simulink model "state_space_all_model_reduce"  (R2018a)
settings: Solver=FixedStepAuto  StartTime=0.0  StopTime=3  FixedStep=tm  MaxStep=1e-4  RelTol=1e-5  AbsTol=1e-5
InitFcn:
  | SimulinkInit_linea_transmision
values from neighbouring files (symbols this model uses):
  Ad = sysd.A    [SimulinkInit_linea_transmision.m]
  ataque = 1    [SimulinkInit_linea_transmision.m]
  b = 4.91    [SimulinkInit_linea_transmision.m]
  Bd = sysd.B    [SimulinkInit_linea_transmision.m]
  Bdr = sysdr.B    [SimulinkInit_linea_transmision.m]
  C = 1    [SimulinkInit_linea_transmision.m]
  C1 = 22e-6    (= 2.2e-05)    [SimulinkInit_linea_transmision.m]
  c11 = 0.04    [SimulinkInit_linea_transmision.m]
  c12 = 0.04    [SimulinkInit_linea_transmision.m]
  c13 = 1.7    [SimulinkInit_linea_transmision.m]
  c14 = 0.17    [SimulinkInit_linea_transmision.m]
  C1o = Cd(2,:)    [SimulinkInit_linea_transmision.m]
  C2 = 22e-6    (= 2.2e-05)    [SimulinkInit_linea_transmision.m]
  c21 = 0.04    [SimulinkInit_linea_transmision.m]
  c22 = 0.04    [SimulinkInit_linea_transmision.m]
  c23 = 1.7    [SimulinkInit_linea_transmision.m]
  c24 = 0.17    [SimulinkInit_linea_transmision.m]
  C2o = Cd(3,:)    [SimulinkInit_linea_transmision.m]
  C3 = 610e-6    (= 0.00061)    [SimulinkInit_linea_transmision.m]
  c31 = 8e-3    (= 0.008)    [SimulinkInit_linea_transmision.m]
  c32 = 0.012    [SimulinkInit_linea_transmision.m]
  c33 = 2.6    [SimulinkInit_linea_transmision.m]
  c34 = 0.24    [SimulinkInit_linea_transmision.m]
  C3o = Cd(4,:)    [SimulinkInit_linea_transmision.m]
  c41 = 0.04    [SimulinkInit_linea_transmision.m]
  c42 = 0.04    [SimulinkInit_linea_transmision.m]
  c43 = 1.7    [SimulinkInit_linea_transmision.m]
  c44 = 0.3    [SimulinkInit_linea_transmision.m]
  C4o = Cd(1,:)    [SimulinkInit_linea_transmision.m]
  Cd = sysd.C    [SimulinkInit_linea_transmision.m]
  Cdr = sysdr.C    [SimulinkInit_linea_transmision.m]
  Cl = 20000e-6    (= 0.02)    [SimulinkInit_linea_transmision.m]
  Jd = 0.3    [SimulinkInit_linea_transmision.m]
  K = 25    [SimulinkInit_linea_transmision.m]    (also in uio_linear.m = K1+E*H)
  K1 = 9.66    [SimulinkInit_linea_transmision.m]    (also in uio_linear.m = K1')
  K11 = 0.8    [SimulinkInit_linea_transmision.m]
  K1d = 1.15    [SimulinkInit_linea_transmision.m]
  K2 = 6.97    [SimulinkInit_linea_transmision.m]
  K22 = 0.2    [SimulinkInit_linea_transmision.m]
  K2d = 1    [SimulinkInit_linea_transmision.m]
  K3 = 31.8    [SimulinkInit_linea_transmision.m]
  K33 = 0.23    [SimulinkInit_linea_transmision.m]
  K3d = 1    [SimulinkInit_linea_transmision.m]
  K4 = 15.1    [SimulinkInit_linea_transmision.m]
  Kd = 0.02    [SimulinkInit_linea_transmision.m]
  Kdc = 0.02    [SimulinkInit_linea_transmision.m]
  Kf = 1    [SimulinkInit_linea_transmision.m]
  Kh = 1.2    [SimulinkInit_linea_transmision.m]
  Ks = 21.5    [SimulinkInit_linea_transmision.m]
  Ksc = 3    [SimulinkInit_linea_transmision.m]
  Kv = 1    [SimulinkInit_linea_transmision.m]
  L = 5.2    [SimulinkInit_linea_transmision.m]
  L1 = 40e-3    (= 0.04)    [SimulinkInit_linea_transmision.m]
  L2 = 30e-3    (= 0.03)    [SimulinkInit_linea_transmision.m]
  L3 = 5e-3    (= 0.005)    [SimulinkInit_linea_transmision.m]
  L4 = 15e-6    (= 1.5e-05)    [SimulinkInit_linea_transmision.m]
  L5 = 12e-6    (= 1.2e-05)    [SimulinkInit_linea_transmision.m]
  L6 = 10e-6    (= 1e-05)    [SimulinkInit_linea_transmision.m]
  Pd = 0.1    [SimulinkInit_linea_transmision.m]
  R = 10    [SimulinkInit_linea_transmision.m]
  R1 = 0.1    [SimulinkInit_linea_transmision.m]
  R2 = 0.2    [SimulinkInit_linea_transmision.m]
  R3 = 1e-3    (= 0.001)    [SimulinkInit_linea_transmision.m]
  R4 = 0.005    [SimulinkInit_linea_transmision.m]
  R5 = 0.0012    [SimulinkInit_linea_transmision.m]
  R6 = .1    (= 0.1)    [SimulinkInit_linea_transmision.m]
  RL = 10    [SimulinkInit_linea_transmision.m]
  Sbin = 13.8    [SimulinkInit_linea_transmision.m]
  sisr = balred(sys,4,opts)    [SimulinkInit_linea_transmision.m]
  Svin = 2.91    [SimulinkInit_linea_transmision.m]
  T1s = 0.4    [SimulinkInit_linea_transmision.m]
  T2s = 1    [SimulinkInit_linea_transmision.m]
  T3s = 15    [SimulinkInit_linea_transmision.m]
  T4s = 2.5    [SimulinkInit_linea_transmision.m]
  T5s = 3.3    [SimulinkInit_linea_transmision.m]
  tao1 = 0.002    [SimulinkInit_linea_transmision.m]
  Tao1d = 0.5    [SimulinkInit_linea_transmision.m]
  tao2 = tao1    (= 0.002)    [SimulinkInit_linea_transmision.m]
  Tao2d = 0.125    [SimulinkInit_linea_transmision.m]
  taod = 1    [SimulinkInit_linea_transmision.m]
  Tcd = 0.2    [SimulinkInit_linea_transmision.m]
  Tcr = 0.01    [SimulinkInit_linea_transmision.m]
  Tf = 0.04    [SimulinkInit_linea_transmision.m]
  tm = 1e-5    (= 1e-05)    [SimulinkInit_linea_transmision.m]
  Tr = 950    [SimulinkInit_linea_transmision.m]
  Tt = 450    [SimulinkInit_linea_transmision.m]
  Ttd = 0.04    [SimulinkInit_linea_transmision.m]
  Tv = 0.05    [SimulinkInit_linea_transmision.m]
  V = 20    [SimulinkInit_linea_transmision.m]
  wref = 70000    [SimulinkInit_linea_transmision.m]
  X_acid = 1.2    [SimulinkInit_linea_transmision.m]
  X_meth = 0.35    [SimulinkInit_linea_transmision.m]
  Z = 3    [SimulinkInit_linea_transmision.m]
undefined symbols (not defined in the file or in its folder): F1, F2, F3, F4, H1, H2, H3, H4, K1U, K2U, K3U, K4U, T1, T2, T3, T4
libraries: neural x277, dsparch4 x4, powerlib_meascontrol x4, mpclib x1, simulink x1
(part 15 of 16)

== system state_space_all_model_reduce/Function Fitting Neural Network4/Layer 2/Delays 1 ==
  "p{2}" : Inport  PortDimensions=30  SampleTime=4e-05
      mask Display: e = 0.06;c1 = [120 230 180]/255;c2 = ([120 230 180]+0)/(256+128);c3 = ([120 230 180]+128)/(256+128);patch([0 1 1 0],[0 0 1 1],c1);patch([0 1 1 1-e 1-e 0+e],[0 0 1 1-e 0+e 0+e],c2);patch([0 0 1 1-e 0+e 0+e],[0 1 1 1-e 1-e 0+e],c3);plot([0 1 1 0 0],[0 0 1 1 0]);
  mux : Mux  Inputs=1
      mask Display: e = 0.06;c1 = [120 150 230]/255;c2 = ([120 150 230]+0)/383;c3 = ([120 150 230]+128)/383;patch([0 1 1 0],[0 0 1 1],c1);patch([0 1 1 1-e 1-e 0+e],[0 0 1 1-e 0+e 0+e],c2);patch([0 0 1 1-e 0+e 0+e],[0 1 1 1-e 1-e 0+e],c3);plot([0 1 1 0 0],[0 0 1 1 0]);disp('Mux')
  "pd{2,1}" : Outport
      mask Display: e = 0.06;c1 = [120 230 180]/255;c2 = ([120 230 180]+0)/(256+128);c3 = ([120 230 180]+128)/(256+128);patch([0 1 1 0],[0 0 1 1],c1);patch([0 1 1 1-e 1-e 0+e],[0 0 1 1-e 0+e 0+e],c2);patch([0 0 1 1-e 0+e 0+e],[0 1 1 1-e 1-e 0+e],c3);plot([0 1 1 0 0],[0 0 1 1 0]);
  wires:
  "p{2}"/1 -> mux/1
  mux/1 -> "pd{2,1}"/1

== system state_space_all_model_reduce/Function Fitting Neural Network4/Layer 2/LW{2,1} ==
  "ad{2,1}" : Inport  PortDimensions=30  SampleTime=4e-05
      mask Display: e = 0.06;c1 = [120 230 180]/255;c2 = ([120 230 180]+0)/(256+128);c3 = ([120 230 180]+128)/(256+128);patch([0 1 1 0],[0 0 1 1],c1);patch([0 1 1 1-e 1-e 0+e],[0 0 1 1-e 0+e 0+e],c2);patch([0 0 1 1-e 0+e 0+e],[0 1 1 1-e 1-e 0+e],c3);plot([0 1 1 0 0],[0 0 1 1 0]);
  "IW{2,1}(1,:)'" : Constant  Value=[0.90714318408745409083593358445796184241771697998046875;-0.048102377339008677015197434911897289566695690155029296875;1.294929042761599813360362531966529786586761474609375;0.206123126824358016140337213073507882654666900634765625;0.45255183578830282531413331525982357561588287353515625;-0.0083287178598355875169811923797169583849608898162841796875;0.51938856593500271063845730168395675718784332275390625;-0.1704080390078703544087801446949015371501445770263671875;0.31513253355746406736415110572124831378459930419921875;0.1800685195147736783471970056780264712870121002197265625;0.37677775106166333518586952777695842087268829345703125;-0.65429506360663591824078366698813624680042266845703125;-0.1459198202949253675431151577868149615824222564697265625;-0.6930340633672076311455612085410393774509429931640625;-0.0265503392239379298889190295085427351295948028564453125;-0.2263814225486771025686039138236083090305328369140625;0.1450935858257641764001988349264138378202915191650390625;-0.42686421614961833626011866726912558078765869140625;0.0140622429623356894057284449672806658782064914703369140625;-0.465063445574494804812815118566504679620265960693359375;-1.352605893942428139098410611040890216827392578125;0.352370261039477827846866375693934969604015350341796875;1.2603949540339789425757999197230674326419830322265625;0.1488977497034494057448483772532199509441852569580078125;1.2975596634931478856600506333052180707454681396484375;0.70692705348580886504095133204828016459941864013671875;-0.36903778142549181762177568089100532233715057373046875;-0.10596122291001329462911684231585240922868251800537109375;0.37083335910809844815361202563508413732051849365234375;0.8086871832562885220596626822953112423419952392578125]
      mask Display: e = 0.06;c1 = [120 150 230]/255;c2 = ([120 150 230]+0)/383;c3 = ([120 150 230]+128)/383;patch([0 1 1 0],[0 0 1 1],c1);patch([0 1 1 1-e 1-e 0+e],[0 0 1 1-e 0+e 0+e],c2);patch([0 0 1 1-e 0+e 0+e],[0 1 1 1-e 1-e 0+e],c3);plot([0 1 1 0 0],[0 0 1 1 0]);disp('weights');
  "IW{2,1}(10,:)'" : Constant  Value=[0.2319138892928117312575153619036427699029445648193359375;-0.8040865402366714764781363555812276899814605712890625;0.9087744071583732097252550374832935631275177001953125;-0.521440952638429155996391273220069706439971923828125;0.60097002100339602659317961297347210347652435302734375;0.36524758320080963347464830803801305592060089111328125;0.1584392130023462019750013496377505362033843994140625;0.1801246098496473158068198472392396070063114166259765625;-0.181406639967756577735968903652974404394626617431640625;-0.296216526047581585334711462564882822334766387939453125;0.312161792653689873500155727015226148068904876708984375;-1.190497919740885368611316152964718639850616455078125;-0.1080333597566015269020311961867264471948146820068359375;1.604326922736868166197155005647800862789154052734375;0.1008958412054597741924766296506277285516262054443359375;-0.97388268375643083363257801465806551277637481689453125;-0.79770811645741102058337901326012797653675079345703125;-0.38900055085768203699814193896600045263767242431640625;-0.384958477415133837329364041579538024961948394775390625;0.11349754296078366777589252478719572536647319793701171875;0.11902848909893372353341334246579208411276340484619140625;0.284680421091827839941146294222562573850154876708984375;1.0325753325713453723011525653419084846973419189453125;0.261504107752342729309447122432175092399120330810546875;-0.794156599441347754719799922895617783069610595703125;0.464018308603296569803120519281947053968906402587890625;-0.630038797774925996009187656454741954803466796875;0.347368201321413827553641340273316018283367156982421875;-0.1174842647443233578652410642462200485169887542724609375;-0.6781726742425444598438843968324363231658935546875]
      mask Display: e = 0.06;c1 = [120 150 230]/255;c2 = ([120 150 230]+0)/383;c3 = ([120 150 230]+128)/383;patch([0 1 1 0],[0 0 1 1],c1);patch([0 1 1 1-e 1-e 0+e],[0 0 1 1-e 0+e 0+e],c2);patch([0 0 1 1-e 0+e 0+e],[0 1 1 1-e 1-e 0+e],c3);plot([0 1 1 0 0],[0 0 1 1 0]);disp('weights');
  "IW{2,1}(2,:)'" : Constant  Value=[0.416947392567051544620682079766993410885334014892578125;0.003266500055877595391773393629364363732747733592987060546875;0.01230846086724191913719383961733910837210714817047119140625;-0.1407463827463234784520551556852296926081180572509765625;0.0122733298540518460939541256493612308986485004425048828125;0.00239388685965834062396861980914763989858329296112060546875;-0.00742694111379034634101703460373755660839378833770751953125;-0.002780624240137022883112560833751558675430715084075927734375;0.000681869839369446330452906313013272665557451546192169189453125;-0.01403327440076230885057650965563880163244903087615966796875;3.648868014078729816833390753316734844702295958995819091796875e-05;0.005269367680551831530089135213756890152581036090850830078125;0.0066467725134027634548150587079362594522535800933837890625;-0.860251710672929714718293325859121978282928466796875;-0.02329516144711478442541618960603955201804637908935546875;-0.006438655230613697134922635001430535339750349521636962890625;0.0267782683650884777148970528060090146027505397796630859375;-0.000530046731904287014326693228127851398312486708164215087890625;0.004411206708843334704794880707368065486662089824676513671875;-0.217414956279098514624337212808313779532909393310546875;0.0028000657909500368224209321255102622671984136104583740234375;-0.003041851155838976202006040949754606117494404315948486328125;-0.06917348842290084454109688749667839147150516510009765625;-0.0190598856354186087236346480722204432822763919830322265625;0.87722079849065714984845953949843533337116241455078125;-0.0053701703131058785289919654815093963406980037689208984375;-0.010446747210423219798247629341858555562794208526611328125;0.000937385564336258385841060825072190709761343896389007568359375;-0.00136150381212682999691743201964300169493071734905242919921875;0.1467966519581848927611389399316976778209209442138671875]
      mask Display: e = 0.06;c1 = [120 150 230]/255;c2 = ([120 150 230]+0)/383;c3 = ([120 150 230]+128)/383;patch([0 1 1 0],[0 0 1 1],c1);patch([0 1 1 1-e 1-e 0+e],[0 0 1 1-e 0+e 0+e],c2);patch([0 0 1 1-e 0+e 0+e],[0 1 1 1-e 1-e 0+e],c3);plot([0 1 1 0 0],[0 0 1 1 0]);disp('weights');
  "IW{2,1}(3,:)'" : Constant  Value=[0.4811326342102930642141700445790775120258331298828125;0.159061399470191988658740456230589188635349273681640625;0.151073188612818209985988460175576619803905487060546875;0.32552722705785541723599862962146289646625518798828125;-0.1601937926922908650428922783248708583414554595947265625;-0.198846871678384273796069692252785898745059967041015625;-0.29414008423258819480139436564058996737003326416015625;0.404441607102767830550504868369898758828639984130859375;-0.0281593321367341886674040551952202804386615753173828125;-0.3874588163011825070469740239786915481090545654296875;0.371708815278716020458205093746073544025421142578125;-0.1359576421882372210259148914701654575765132904052734375;-0.291217292857733955901977651592460460960865020751953125;-0.330039596205321306143787296605296432971954345703125;0.043988003155176168268436498465234762988984584808349609375;0.030546221792962346963662412235862575471401214599609375;0.0024517022889222173619161448954173465608619153499603271484375;0.08799926141388014766420155865489505231380462646484375;-0.0252825080093841240980179208008848945610225200653076171875;-0.0172303460256001128581004877560189925134181976318359375;0.2085776997870492921460794377708225511014461517333984375;-0.11072455894766426720554619578251731581985950469970703125;-1.32223818855680352868375848629511892795562744140625;-0.2884710339757681207828454716945998370647430419921875;0.542892688510505205812251006136648356914520263671875;0.1253472561014621067254637409860151819884777069091796875;-0.2529193370139160013110313229844905436038970947265625;-0.1616420982781887338841642076658899895846843719482421875;-0.344729343588641878870504342557978816330432891845703125;0.32437295849790925839073452152661047875881195068359375]
      mask Display: e = 0.06;c1 = [120 150 230]/255;c2 = ([120 150 230]+0)/383;c3 = ([120 150 230]+128)/383;patch([0 1 1 0],[0 0 1 1],c1);patch([0 1 1 1-e 1-e 0+e],[0 0 1 1-e 0+e 0+e],c2);patch([0 0 1 1-e 0+e 0+e],[0 1 1 1-e 1-e 0+e],c3);plot([0 1 1 0 0],[0 0 1 1 0]);disp('weights');
  "IW{2,1}(4,:)'" : Constant  Value=[0.780427241542826610753991189994849264621734619140625;0.057530472678189191471087582385735004208981990814208984375;-0.51241431532391745751198186553665436804294586181640625;-0.76645255461915040573472879259497858583927154541015625;0.49550525807477452389093741658143699169158935546875;-0.496561259751099048909139810348278842866420745849609375;-1.5466382185052955922088813167647458612918853759765625;0.284340016361476821682430227156146429479122161865234375;0.0267426142921908006899744947304498055018484592437744140625;1.012097772063371703410439295112155377864837646484375;-0.1260666622690852223254154296228080056607723236083984375;-0.344162807623067334983346654553315602242946624755859375;0.44401932774356211997002219504793174564838409423828125;0.291297046140281679083017252196441404521465301513671875;0.276736552166026050780800460415775887668132781982421875;-0.0627395377176816204656262243588571436703205108642578125;-0.8076630578576164953830129888956435024738311767578125;0.13742217281169388787276375296642072498798370361328125;-0.1653909969925929923650897990228259004652500152587890625;0.7811361009917618947184791977633722126483917236328125;-0.181846525580031947999515296032768674194812774658203125;0.440317068787857424094767111455439589917659759521484375;-0.65945057493641934254213765598251484334468841552734375;-0.65340363329524009383675320350448600947856903076171875;-0.3663726476927198216770875660586170852184295654296875;0.09270976273430819869503238805918954312801361083984375;-0.6874958771821422232051190803758800029754638671875;-0.112275761061875256618947105380357243120670318603515625;-0.2102619194012265435578257211091113276779651641845703125;-0.253371286235020753974112039941246621310710906982421875]
      mask Display: e = 0.06;c1 = [120 150 230]/255;c2 = ([120 150 230]+0)/383;c3 = ([120 150 230]+128)/383;patch([0 1 1 0],[0 0 1 1],c1);patch([0 1 1 1-e 1-e 0+e],[0 0 1 1-e 0+e 0+e],c2);patch([0 0 1 1-e 0+e 0+e],[0 1 1 1-e 1-e 0+e],c3);plot([0 1 1 0 0],[0 0 1 1 0]);disp('weights');
  "IW{2,1}(5,:)'" : Constant  Value=[-0.50117042530569555491837263616616837680339813232421875;-0.0039021865824777177307602915590223346953280270099639892578125;-0.01473480686419767309025541379696733201853930950164794921875;-1.0968451686606386363820320184458978474140167236328125;-0.01482478007369248708402498238001498975791037082672119140625;-0.002776499863896996454781795904409591457806527614593505859375;0.00901481535869287468887289804797546821646392345428466796875;0.0032980166278300700188896854569975403137505054473876953125;-0.000849023211864692096441376012450064081349410116672515869140625;0.01696999705323133655898715232979157008230686187744140625;-4.0593417078821047148419476346958845169865526258945465087890625e-05;-0.00635490758808683782465909217762600746937096118927001953125;-0.0079831878148326380906230070877427351661026477813720703125;-0.497153347444955817646672358023351989686489105224609375;0.028066631642862875650745735356395016424357891082763671875;0.007705945839800311392142617705758311785757541656494140625;-0.032322189165419325240780068497770116664469242095947265625;0.00060982541674404057256697608835338542121462523937225341796875;-0.005289089408298701562582966317904720199294388294219970703125;0.2619989696036253423727657718700356781482696533203125;-0.0033771084089689357328467611552014204789884388446807861328125;0.003723948646043295611363088681855515460483729839324951171875;0.0829829244235045226929514683433808386325836181640625;0.0228557795202047088489738513317206525243818759918212890625;0.6316288380182248918259801939711906015872955322265625;0.006427797332537212027236961375820101238787174224853515625;0.012594311678557450207005530273818294517695903778076171875;-0.001068075378483649730265714339338956051506102085113525390625;0.0016306720221492608351165909397195719066075980663299560546875;-0.1761434736558893376923151663504540920257568359375]
      mask Display: e = 0.06;c1 = [120 150 230]/255;c2 = ([120 150 230]+0)/383;c3 = ([120 150 230]+128)/383;patch([0 1 1 0],[0 0 1 1],c1);patch([0 1 1 1-e 1-e 0+e],[0 0 1 1-e 0+e 0+e],c2);patch([0 0 1 1-e 0+e 0+e],[0 1 1 1-e 1-e 0+e],c3);plot([0 1 1 0 0],[0 0 1 1 0]);disp('weights');
  "IW{2,1}(6,:)'" : Constant  Value=[0.7896233319836287734005964011885225772857666015625;-0.60868667462329428818890164620825089514255523681640625;1.0936294370899932726359793377923779189586639404296875;-0.6712363747772684963166511806775815784931182861328125;-0.526223852964790683728324438561685383319854736328125;-0.1607090820942050080066820783031289465725421905517578125;-0.626106869773626062425364580121822655200958251953125;0.06496541718792249453517939628000021912157535552978515625;0.83610720276940408979271524003706872463226318359375;-0.6929388325834029416228077025152742862701416015625;-1.067185172155014516448545691673643887042999267578125;0.52897399748873474845112241382594220340251922607421875;-0.25044795144986886636928602456464432179927825927734375;2.693622832879899231528497693943791091442108154296875;-0.07305148165279219674150823493619100190699100494384765625;-0.493246738666023976094265890424139797687530517578125;0.4335866046076308766288320839521475136280059814453125;-0.3897028848922257093789767168345861136913299560546875;0.5841730845356003509749598379130475223064422607421875;-0.421691298090711430557320227308082394301891326904296875;0.6227543394190220293893389680306427180767059326171875;-0.7864576605892763527805300327599979937076568603515625;1.4226306632008440811176797069492749869823455810546875;-1.1047050983499018261824176079244352877140045166015625;0.129955616195306600246794914710335433483123779296875;0.8838242332930856814954267974826507270336151123046875;-0.06430126068878465328548799107011291198432445526123046875;0.1257806812499334958577179577332572080194950103759765625;0.2426547734963307723088377088060951791703701019287109375;0.002085020601967785443264791211959163774736225605010986328125]
      mask Display: e = 0.06;c1 = [120 150 230]/255;c2 = ([120 150 230]+0)/383;c3 = ([120 150 230]+128)/383;patch([0 1 1 0],[0 0 1 1],c1);patch([0 1 1 1-e 1-e 0+e],[0 0 1 1-e 0+e 0+e],c2);patch([0 0 1 1-e 0+e 0+e],[0 1 1 1-e 1-e 0+e],c3);plot([0 1 1 0 0],[0 0 1 1 0]);disp('weights');
  "IW{2,1}(7,:)'" : Constant  Value=[0.04309644542072887940520331540028564631938934326171875;0.168206520815998794571299868039204739034175872802734375;-0.483876365756592097255861517623998224735260009765625;-0.421792672787994593619487204705365002155303955078125;-0.0981928047716486840368332877915236167609691619873046875;-0.55992626237072806727468332610442303121089935302734375;0.2336871391025230615401397926689242012798786163330078125;-0.152405391462436312632888757434557192027568817138671875;0.295437518929980214021924211920122615993022918701171875;0.09530249896765095873885087485177791677415370941162109375;-0.22891937209391433061256293512997217476367950439453125;0.2282840336826637284151075846239109523594379425048828125;-0.92474127052569254914260454825125634670257568359375;1.548429152866563018875467605539597570896148681640625;-0.74378969042484721629904242945485748350620269775390625;0.1626424687577106009683802767540328204631805419921875;-0.608083672851356116240140181616879999637603759765625;-0.01014717518381154891249362748339990503154695034027099609375;0.16256722480110408213249684195034205913543701171875;-1.1432129069102059393259196440340019762516021728515625;-0.01207813138522211525438532220277920714579522609710693359375;0.9454535378756403485311921031097881495952606201171875;0.2049811662502954712206104659344418905675411224365234375;0.0032446575932436653132151516132353208377026021480560302734375;-0.207132310225231985878480145402136258780956268310546875;0.343946835770849668190152215174748562276363372802734375;-0.278827129264008544140551748569123446941375732421875;-0.035871968458857643458070896258504944853484630584716796875;0.7674182727494989197936092750751413404941558837890625;-0.35772812559392974662841879762709140777587890625]
      mask Display: e = 0.06;c1 = [120 150 230]/255;c2 = ([120 150 230]+0)/383;c3 = ([120 150 230]+128)/383;patch([0 1 1 0],[0 0 1 1],c1);patch([0 1 1 1-e 1-e 0+e],[0 0 1 1-e 0+e 0+e],c2);patch([0 0 1 1-e 0+e 0+e],[0 1 1 1-e 1-e 0+e],c3);plot([0 1 1 0 0],[0 0 1 1 0]);disp('weights');
  "IW{2,1}(8,:)'" : Constant  Value=[-0.1353297288916197882446823541613412089645862579345703125;-0.0216029369393972402180192915466250269673764705657958984375;0.2007551311806741178855872931308113038539886474609375;-0.64722103301441114009406874174601398408412933349609375;0.12265007064435555494963381306661176495254039764404296875;-0.97005846783641846986512291550752706825733184814453125;-0.52928964999073946362528886311338283121585845947265625;-0.08745241800787910413372827633793349377810955047607421875;0.7727495405352018398303926005610264837741851806640625;-0.486770003641608883793168160991626791656017303466796875;-0.0338725998204997547080807862585061229765415191650390625;0.67068681412624953086520918077440001070499420166015625;-0.480647470994034708979825154528953135013580322265625;-2.0054703998628209404841982177458703517913818359375;0.72507447780183775787321565076126717031002044677734375;0.90018682212346290416604688289226032793521881103515625;0.13235978028933137462530567063367925584316253662109375;1.1950727805776413248395328992046415805816650390625;0.1923213227530198021764107352282735519111156463623046875;1.1236929112923821350022990372963249683380126953125;-0.0606041823980134619631598980049602687358856201171875;-0.1036887637510263415752120863544405438005924224853515625;-0.69702032678725955872067743257503025233745574951171875;0.57154667176720475030293755480670370161533355712890625;-0.726454909640519730373853235505521297454833984375;-0.323668732683641879877001201748498715460300445556640625;-0.12087904607715671545520308427512645721435546875;-0.5995296715433087175739501617499627172946929931640625;-0.401740924345518390925491303278249688446521759033203125;-0.9087221222252244157147060832357965409755706787109375]
      mask Display: e = 0.06;c1 = [120 150 230]/255;c2 = ([120 150 230]+0)/383;c3 = ([120 150 230]+128)/383;patch([0 1 1 0],[0 0 1 1],c1);patch([0 1 1 1-e 1-e 0+e],[0 0 1 1-e 0+e 0+e],c2);patch([0 0 1 1-e 0+e 0+e],[0 1 1 1-e 1-e 0+e],c3);plot([0 1 1 0 0],[0 0 1 1 0]);disp('weights');
  "IW{2,1}(9,:)'" : Constant  Value=[0.47379853716004716179810429821372963488101959228515625;-0.406311319271628390570327837849617935717105865478515625;0.5259855644641360239432970047346316277980804443359375;-1.1216862632571948932280747612821869552135467529296875;-0.316968682311370042459230944587034173309803009033203125;-0.65720087833227081031139960032305680215358734130859375;0.455612594975877971403832589203375391662120819091796875;0.337814812302101474816851123250671662390232086181640625;0.4476635194369453785157020320184528827667236328125;-0.07322083945893607948018910747123300097882747650146484375;-0.335521835144620583779584421790787018835544586181640625;0.47289311293118674317526028971769846975803375244140625;-0.48635063495489838647500846491311676800251007080078125;0.9643117682098159004766557700349949300289154052734375;-0.912602132425770928847441609832458198070526123046875;1.2500845871907444450954471903969533741474151611328125;0.061872709894893684889893847866915166378021240234375;0.764083959372054533076834559324197471141815185546875;0.452783356866307773458402152755297720432281494140625;-0.38881286148172045091797599525307305157184600830078125;-0.13196645046089716668546998334932141005992889404296875;0.482531389258949505727258610932040028274059295654296875;0.230617361345195781563433001792873255908489227294921875;-0.57245066329090110723853968011098913848400115966796875;0.04650247124085714334196239860830246470868587493896484375;-1.067909673790131019899263264960609376430511474609375;0.299393463266107051623521329020150005817413330078125;0.004515326929721389347116566881368271424435079097747802734375;1.0745421262124212891109209522255696356296539306640625;-0.20141470927993143646972384885884821414947509765625]
      mask Display: e = 0.06;c1 = [120 150 230]/255;c2 = ([120 150 230]+0)/383;c3 = ([120 150 230]+128)/383;patch([0 1 1 0],[0 0 1 1],c1);patch([0 1 1 1-e 1-e 0+e],[0 0 1 1-e 0+e 0+e],c2);patch([0 0 1 1-e 0+e 0+e],[0 1 1 1-e 1-e 0+e],c3);plot([0 1 1 0 0],[0 0 1 1 0]);disp('weights');
  Mux : Mux  Inputs=10
      mask Display: e = 0.06;c1 = [120 150 230]/255;c2 = ([120 150 230]+0)/383;c3 = ([120 150 230]+128)/383;patch([0 1 1 0],[0 0 1 1],c1);patch([0 1 1 1-e 1-e 0+e],[0 0 1 1-e 0+e 0+e],c2);patch([0 0 1 1-e 0+e 0+e],[0 1 1 1-e 1-e 0+e],c3);plot([0 1 1 0 0],[0 0 1 1 0]);disp('Mux');
  dotprod{1..10} (10 alike) : neural/Weight Functions/dotprod
  "lz{2,1}" : Outport
      mask Display: e = 0.06;c1 = [120 230 180]/255;c2 = ([120 230 180]+0)/(256+128);c3 = ([120 230 180]+128)/(256+128);patch([0 1 1 0],[0 0 1 1],c1);patch([0 1 1 1-e 1-e 0+e],[0 0 1 1-e 0+e 0+e],c2);patch([0 0 1 1-e 0+e 0+e],[0 1 1 1-e 1-e 0+e],c3);plot([0 1 1 0 0],[0 0 1 1 0]);
  wires:
  "IW{2,1}(1,:)'"/1 -> dotprod1/1
  "ad{2,1}"/1 -> dotprod1/2, dotprod2/2, dotprod3/2, dotprod4/2, dotprod5/2, dotprod6/2, dotprod7/2, dotprod8/2, dotprod9/2, dotprod10/2
  dotprod1/1 -> Mux/1
  "IW{2,1}(2,:)'"/1 -> dotprod2/1
  dotprod2/1 -> Mux/2
  "IW{2,1}(3,:)'"/1 -> dotprod3/1
  dotprod3/1 -> Mux/3
  "IW{2,1}(4,:)'"/1 -> dotprod4/1
  dotprod4/1 -> Mux/4
  "IW{2,1}(5,:)'"/1 -> dotprod5/1
  dotprod5/1 -> Mux/5
  "IW{2,1}(6,:)'"/1 -> dotprod6/1
  dotprod6/1 -> Mux/6
  "IW{2,1}(7,:)'"/1 -> dotprod7/1
  dotprod7/1 -> Mux/7
  "IW{2,1}(8,:)'"/1 -> dotprod8/1
  dotprod8/1 -> Mux/8
  "IW{2,1}(9,:)'"/1 -> dotprod9/1
  dotprod9/1 -> Mux/9
  "IW{2,1}(10,:)'"/1 -> dotprod10/1
  dotprod10/1 -> Mux/10
  Mux/1 -> "lz{2,1}"/1

== system state_space_all_model_reduce/Function Fitting Neural Network4/Layer 3/Delays 1 ==
  "p{3}" : Inport  PortDimensions=10  SampleTime=4e-05
      mask Display: e = 0.06;c1 = [120 230 180]/255;c2 = ([120 230 180]+0)/(256+128);c3 = ([120 230 180]+128)/(256+128);patch([0 1 1 0],[0 0 1 1],c1);patch([0 1 1 1-e 1-e 0+e],[0 0 1 1-e 0+e 0+e],c2);patch([0 0 1 1-e 0+e 0+e],[0 1 1 1-e 1-e 0+e],c3);plot([0 1 1 0 0],[0 0 1 1 0]);
  mux : Mux  Inputs=1
      mask Display: e = 0.06;c1 = [120 150 230]/255;c2 = ([120 150 230]+0)/383;c3 = ([120 150 230]+128)/383;patch([0 1 1 0],[0 0 1 1],c1);patch([0 1 1 1-e 1-e 0+e],[0 0 1 1-e 0+e 0+e],c2);patch([0 0 1 1-e 0+e 0+e],[0 1 1 1-e 1-e 0+e],c3);plot([0 1 1 0 0],[0 0 1 1 0]);disp('Mux')
  "pd{3,2}" : Outport
      mask Display: e = 0.06;c1 = [120 230 180]/255;c2 = ([120 230 180]+0)/(256+128);c3 = ([120 230 180]+128)/(256+128);patch([0 1 1 0],[0 0 1 1],c1);patch([0 1 1 1-e 1-e 0+e],[0 0 1 1-e 0+e 0+e],c2);patch([0 0 1 1-e 0+e 0+e],[0 1 1 1-e 1-e 0+e],c3);plot([0 1 1 0 0],[0 0 1 1 0]);
  wires:
  "p{3}"/1 -> mux/1
  mux/1 -> "pd{3,2}"/1

== system state_space_all_model_reduce/Function Fitting Neural Network4/Layer 3/LW{3,2} ==
  "ad{3,2}" : Inport  PortDimensions=10  SampleTime=4e-05
      mask Display: e = 0.06;c1 = [120 230 180]/255;c2 = ([120 230 180]+0)/(256+128);c3 = ([120 230 180]+128)/(256+128);patch([0 1 1 0],[0 0 1 1],c1);patch([0 1 1 1-e 1-e 0+e],[0 0 1 1-e 0+e 0+e],c2);patch([0 0 1 1-e 0+e 0+e],[0 1 1 1-e 1-e 0+e],c3);plot([0 1 1 0 0],[0 0 1 1 0]);
  "IW{3,2}(1,:)'" : Constant  Value=[0.9710363259008365499624915173626504838466644287109375;-2.51187609213334805957629214390181005001068115234375;-1.1754207675500207841423616628162562847137451171875;-1.977263433643422718688498207484371960163116455078125;1.1382477731081299676674234433448873460292816162109375;0.39457203162995024836590118866297416388988494873046875;1.163142847407714786100996207096613943576812744140625;-0.19765672112898735601760336066945455968379974365234375;0.537743359369233342448524126666598021984100341796875;2.1099403819780189195398634183220565319061279296875]
      mask Display: e = 0.06;c1 = [120 150 230]/255;c2 = ([120 150 230]+0)/383;c3 = ([120 150 230]+128)/383;patch([0 1 1 0],[0 0 1 1],c1);patch([0 1 1 1-e 1-e 0+e],[0 0 1 1-e 0+e 0+e],c2);patch([0 0 1 1-e 0+e 0+e],[0 1 1 1-e 1-e 0+e],c3);plot([0 1 1 0 0],[0 0 1 1 0]);disp('weights');
  "IW{3,2}(10,:)'" : Constant  Value=[-0.1945340597322998965612583788242773152887821197509765625;0.763677470190639695601930725388228893280029296875;1.0597926224578932963282795753912068903446197509765625;0.262445300397221803478942092624492943286895751953125;-1.4355254388695606326820097820018418133258819580078125;0.0281593561954353970022690845098622958175837993621826171875;-0.31688095645483638218564692579093389213085174560546875;0.07638317313643848416315762506201281212270259857177734375;0.0019591936009257025601282276028314299765042960643768310546875;-1.310982766706533464429185187327675521373748779296875]
      mask Display: e = 0.06;c1 = [120 150 230]/255;c2 = ([120 150 230]+0)/383;c3 = ([120 150 230]+128)/383;patch([0 1 1 0],[0 0 1 1],c1);patch([0 1 1 1-e 1-e 0+e],[0 0 1 1-e 0+e 0+e],c2);patch([0 0 1 1-e 0+e 0+e],[0 1 1 1-e 1-e 0+e],c3);plot([0 1 1 0 0],[0 0 1 1 0]);disp('weights');
  "IW{3,2}(2,:)'" : Constant  Value=[1.8794364067859270495119972110842354595661163330078125;0.7856775240973068452632332991925068199634552001953125;1.1393970149721026619005215252400375902652740478515625;-2.1250049371964667699330675532110035419464111328125;-1.01263647334854312020979705266654491424560546875;0.501468496372924565918083317228592932224273681640625;-0.9027735833732626336001203526393510401248931884765625;0.3728696196779097693507765143294818699359893798828125;-1.5842264243608565887910799574456177651882171630859375;-0.743445294339208029299470581463538110256195068359375]
      mask Display: e = 0.06;c1 = [120 150 230]/255;c2 = ([120 150 230]+0)/383;c3 = ([120 150 230]+128)/383;patch([0 1 1 0],[0 0 1 1],c1);patch([0 1 1 1-e 1-e 0+e],[0 0 1 1-e 0+e 0+e],c2);patch([0 0 1 1-e 0+e 0+e],[0 1 1 1-e 1-e 0+e],c3);plot([0 1 1 0 0],[0 0 1 1 0]);disp('weights');
  "IW{3,2}(3,:)'" : Constant  Value=[-0.43119967227037514501120085697039030492305755615234375;0.36674847139058919243126410947297699749469757080078125;1.7469204420679622646872530822292901575565338134765625;1.598890628958684612115348500083200633525848388671875;-0.5628842447266582116327526819077320396900177001953125;-0.77423277129793943718283344423980452120304107666015625;-0.45869032098220030579938111259252764284610748291015625;-0.27057509026289061626613374755834229290485382080078125;-1.438764134822528628632198888226412236690521240234375;-1.1699285966508752299120033057988621294498443603515625]
      mask Display: e = 0.06;c1 = [120 150 230]/255;c2 = ([120 150 230]+0)/383;c3 = ([120 150 230]+128)/383;patch([0 1 1 0],[0 0 1 1],c1);patch([0 1 1 1-e 1-e 0+e],[0 0 1 1-e 0+e 0+e],c2);patch([0 0 1 1-e 0+e 0+e],[0 1 1 1-e 1-e 0+e],c3);plot([0 1 1 0 0],[0 0 1 1 0]);disp('weights');
  "IW{3,2}(4,:)'" : Constant  Value=[-0.017818140574946440823911331108320155180990695953369140625;-0.6088580158768228667298672007746063172817230224609375;-0.03267000336322321840665239278678200207650661468505859375;-0.023870405366698134452807522620787494815886020660400390625;-0.640631893012377329199580344720743596553802490234375;0.0031630676749337355117830394846123454044573009014129638671875;0.0374790806375362717250965260973316617310047149658203125;-0.018264798522163956662200945402219076640903949737548828125;-0.0030833678587255798457522626421223321813158690929412841796875;0.034572627397432727225368154222451266832649707794189453125]
      mask Display: e = 0.06;c1 = [120 150 230]/255;c2 = ([120 150 230]+0)/383;c3 = ([120 150 230]+128)/383;patch([0 1 1 0],[0 0 1 1],c1);patch([0 1 1 1-e 1-e 0+e],[0 0 1 1-e 0+e 0+e],c2);patch([0 0 1 1-e 0+e 0+e],[0 1 1 1-e 1-e 0+e],c3);plot([0 1 1 0 0],[0 0 1 1 0]);disp('weights');
  "IW{3,2}(5,:)'" : Constant  Value=[0.01511042964432748013370311213066088384948670864105224609375;-1.1105971862212944412107162861502729356288909912109375;0.08187355184278853614809889904790907166898250579833984375;0.0171823921856681556541435185181398992426693439483642578125;-0.68920654712249540541080250477534718811511993408203125;-0.00336178538255475604923372401344749960117042064666748046875;-0.026689692918703468438312853550087311305105686187744140625;0.020278538145916187585005019400341552682220935821533203125;0.0033463234392501401727459953150400906451977789402008056640625;-0.01524475588461773369053364746150691644288599491119384765625]
      mask Display: e = 0.06;c1 = [120 150 230]/255;c2 = ([120 150 230]+0)/383;c3 = ([120 150 230]+128)/383;patch([0 1 1 0],[0 0 1 1],c1);patch([0 1 1 1-e 1-e 0+e],[0 0 1 1-e 0+e 0+e],c2);patch([0 0 1 1-e 0+e 0+e],[0 1 1 1-e 1-e 0+e],c3);plot([0 1 1 0 0],[0 0 1 1 0]);disp('weights');
  "IW{3,2}(6,:)'" : Constant  Value=[-0.005830212846177656137169886818583108833990991115570068359375;-0.1664485302442659520050227683896082453429698944091796875;0.72462924944036355423548911858233623206615447998046875;-0.046582911489240215463514260818556067533791065216064453125;1.4620438118241263492080861396971158683300018310546875;-0.00836081878249448316731129438039715751074254512786865234375;0.077283554294248546501222563165356405079364776611328125;0.061163431162863483858682656091332319192588329315185546875;0.00875328484770362784395114630342504824511706829071044921875;0.1934686481773077171286701059216284193098545074462890625]
      mask Display: e = 0.06;c1 = [120 150 230]/255;c2 = ([120 150 230]+0)/383;c3 = ([120 150 230]+128)/383;patch([0 1 1 0],[0 0 1 1],c1);patch([0 1 1 1-e 1-e 0+e],[0 0 1 1-e 0+e 0+e],c2);patch([0 0 1 1-e 0+e 0+e],[0 1 1 1-e 1-e 0+e],c3);plot([0 1 1 0 0],[0 0 1 1 0]);disp('weights');
  "IW{3,2}(7,:)'" : Constant  Value=[1.0567466340260367463343982308288104832172393798828125;0.1427357264153042704091234327279380522668361663818359375;-1.6608711852453534874030083301477134227752685546875;1.306512482367690797246950751286931335926055908203125;-2.39683135086531340363080744282342493534088134765625;-0.259854129397881161711580944029265083372592926025390625;-0.413502192224532716391394160382333211600780487060546875;1.7695072600376253735277032319572754204273223876953125;-1.462095749593834259627556093619205057621002197265625;0.0912433972384120439702570592999109067022800445556640625]
      mask Display: e = 0.06;c1 = [120 150 230]/255;c2 = ([120 150 230]+0)/383;c3 = ([120 150 230]+128)/383;patch([0 1 1 0],[0 0 1 1],c1);patch([0 1 1 1-e 1-e 0+e],[0 0 1 1-e 0+e 0+e],c2);patch([0 0 1 1-e 0+e 0+e],[0 1 1 1-e 1-e 0+e],c3);plot([0 1 1 0 0],[0 0 1 1 0]);disp('weights');
  "IW{3,2}(8,:)'" : Constant  Value=[0.1877223994986507438209599740730482153594493865966796875;1.0521267722207572337111969318357296288013458251953125;-1.8904523427806647628557357165846042335033416748046875;0.1233197802213740479349013412502245046198368072509765625;-0.2060629622286287709886920538338017649948596954345703125;0.0797888805049830340809791096035041846334934234619140625;0.1418728020708309445208072929744957946240901947021484375;-0.56314700590606048269393113514524884521961212158203125;0.10373536894603858915520078198824194259941577911376953125;0.16286365014989934163480711504234932363033294677734375]
      mask Display: e = 0.06;c1 = [120 150 230]/255;c2 = ([120 150 230]+0)/383;c3 = ([120 150 230]+128)/383;patch([0 1 1 0],[0 0 1 1],c1);patch([0 1 1 1-e 1-e 0+e],[0 0 1 1-e 0+e 0+e],c2);patch([0 0 1 1-e 0+e 0+e],[0 1 1 1-e 1-e 0+e],c3);plot([0 1 1 0 0],[0 0 1 1 0]);disp('weights');
  "IW{3,2}(9,:)'" : Constant  Value=[0.51198877926697716755910505526117049157619476318359375;0.68774971776655380306664255840587429702281951904296875;1.1535131876574951093061827123165130615234375;0.160297297442587360905008608824573457241058349609375;0.335448400712621996877516039603506214916706085205078125;-0.1456873009959310516503450116942985914647579193115234375;0.470397604828699134049685426361975260078907012939453125;-0.0092218959113650016135022013941124896518886089324951171875;-0.337876024197187152520172048753011040389537811279296875;0.044870633097728061799980281421085237525403499603271484375]
      mask Display: e = 0.06;c1 = [120 150 230]/255;c2 = ([120 150 230]+0)/383;c3 = ([120 150 230]+128)/383;patch([0 1 1 0],[0 0 1 1],c1);patch([0 1 1 1-e 1-e 0+e],[0 0 1 1-e 0+e 0+e],c2);patch([0 0 1 1-e 0+e 0+e],[0 1 1 1-e 1-e 0+e],c3);plot([0 1 1 0 0],[0 0 1 1 0]);disp('weights');
  Mux : Mux  Inputs=10
      mask Display: e = 0.06;c1 = [120 150 230]/255;c2 = ([120 150 230]+0)/383;c3 = ([120 150 230]+128)/383;patch([0 1 1 0],[0 0 1 1],c1);patch([0 1 1 1-e 1-e 0+e],[0 0 1 1-e 0+e 0+e],c2);patch([0 0 1 1-e 0+e 0+e],[0 1 1 1-e 1-e 0+e],c3);plot([0 1 1 0 0],[0 0 1 1 0]);disp('Mux');
  dotprod{1..10} (10 alike) : neural/Weight Functions/dotprod
  "lz{3,2}" : Outport
      mask Display: e = 0.06;c1 = [120 230 180]/255;c2 = ([120 230 180]+0)/(256+128);c3 = ([120 230 180]+128)/(256+128);patch([0 1 1 0],[0 0 1 1],c1);patch([0 1 1 1-e 1-e 0+e],[0 0 1 1-e 0+e 0+e],c2);patch([0 0 1 1-e 0+e 0+e],[0 1 1 1-e 1-e 0+e],c3);plot([0 1 1 0 0],[0 0 1 1 0]);
  wires:
  "IW{3,2}(1,:)'"/1 -> dotprod1/1
  "ad{3,2}"/1 -> dotprod1/2, dotprod2/2, dotprod3/2, dotprod4/2, dotprod5/2, dotprod6/2, dotprod7/2, dotprod8/2, dotprod9/2, dotprod10/2
  dotprod1/1 -> Mux/1
  "IW{3,2}(2,:)'"/1 -> dotprod2/1
  dotprod2/1 -> Mux/2
  "IW{3,2}(3,:)'"/1 -> dotprod3/1
  dotprod3/1 -> Mux/3
  "IW{3,2}(4,:)'"/1 -> dotprod4/1
  dotprod4/1 -> Mux/4
  "IW{3,2}(5,:)'"/1 -> dotprod5/1
  dotprod5/1 -> Mux/5
  "IW{3,2}(6,:)'"/1 -> dotprod6/1
  dotprod6/1 -> Mux/6
  "IW{3,2}(7,:)'"/1 -> dotprod7/1
  dotprod7/1 -> Mux/7
  "IW{3,2}(8,:)'"/1 -> dotprod8/1
  dotprod8/1 -> Mux/8
  "IW{3,2}(9,:)'"/1 -> dotprod9/1
  dotprod9/1 -> Mux/9
  "IW{3,2}(10,:)'"/1 -> dotprod10/1
  dotprod10/1 -> Mux/10
  Mux/1 -> "lz{3,2}"/1

== system state_space_all_model_reduce/Function Fitting Neural Network4/Layer 4/Delays 1 ==
  "p{4}" : Inport  PortDimensions=10  SampleTime=4e-05
      mask Display: e = 0.06;c1 = [120 230 180]/255;c2 = ([120 230 180]+0)/(256+128);c3 = ([120 230 180]+128)/(256+128);patch([0 1 1 0],[0 0 1 1],c1);patch([0 1 1 1-e 1-e 0+e],[0 0 1 1-e 0+e 0+e],c2);patch([0 0 1 1-e 0+e 0+e],[0 1 1 1-e 1-e 0+e],c3);plot([0 1 1 0 0],[0 0 1 1 0]);
  mux : Mux  Inputs=1
      mask Display: e = 0.06;c1 = [120 150 230]/255;c2 = ([120 150 230]+0)/383;c3 = ([120 150 230]+128)/383;patch([0 1 1 0],[0 0 1 1],c1);patch([0 1 1 1-e 1-e 0+e],[0 0 1 1-e 0+e 0+e],c2);patch([0 0 1 1-e 0+e 0+e],[0 1 1 1-e 1-e 0+e],c3);plot([0 1 1 0 0],[0 0 1 1 0]);disp('Mux')
  "pd{4,3}" : Outport
      mask Display: e = 0.06;c1 = [120 230 180]/255;c2 = ([120 230 180]+0)/(256+128);c3 = ([120 230 180]+128)/(256+128);patch([0 1 1 0],[0 0 1 1],c1);patch([0 1 1 1-e 1-e 0+e],[0 0 1 1-e 0+e 0+e],c2);patch([0 0 1 1-e 0+e 0+e],[0 1 1 1-e 1-e 0+e],c3);plot([0 1 1 0 0],[0 0 1 1 0]);
  wires:
  "p{4}"/1 -> mux/1
  mux/1 -> "pd{4,3}"/1

== system state_space_all_model_reduce/Function Fitting Neural Network4/Layer 4/LW{4,3} ==
  "ad{4,3}" : Inport  PortDimensions=10  SampleTime=4e-05
      mask Display: e = 0.06;c1 = [120 230 180]/255;c2 = ([120 230 180]+0)/(256+128);c3 = ([120 230 180]+128)/(256+128);patch([0 1 1 0],[0 0 1 1],c1);patch([0 1 1 1-e 1-e 0+e],[0 0 1 1-e 0+e 0+e],c2);patch([0 0 1 1-e 0+e 0+e],[0 1 1 1-e 1-e 0+e],c3);plot([0 1 1 0 0],[0 0 1 1 0]);
  "IW{4,3}(1,:)'" : Constant  Value=[-9.2585086247419791610595296571517565098474733531475067138671875e-06;-1.847341501796418244377324946459140164733980782330036163330078125e-05;-2.614673865195694184532064496817582721632788889110088348388671875e-05;-1.9295132245544210913834604070871137082576751708984375;-2.22021580019332187561076352722011506557464599609375;0.1686040578134969381007834954289137385785579681396484375;1.2869175278299053308207929025019922164574381895363330841064453125e-05;0.50721165726281725039115144682000391185283660888671875;2.085269152762117639905888044626891542066005058586597442626953125e-05;-0.00060853082162002605955131162573934489046223461627960205078125]
      mask Display: e = 0.06;c1 = [120 150 230]/255;c2 = ([120 150 230]+0)/383;c3 = ([120 150 230]+128)/383;patch([0 1 1 0],[0 0 1 1],c1);patch([0 1 1 1-e 1-e 0+e],[0 0 1 1-e 0+e 0+e],c2);patch([0 0 1 1-e 0+e 0+e],[0 1 1 1-e 1-e 0+e],c3);plot([0 1 1 0 0],[0 0 1 1 0]);disp('weights');
  Mux : Mux  Inputs=1
      mask Display: e = 0.06;c1 = [120 150 230]/255;c2 = ([120 150 230]+0)/383;c3 = ([120 150 230]+128)/383;patch([0 1 1 0],[0 0 1 1],c1);patch([0 1 1 1-e 1-e 0+e],[0 0 1 1-e 0+e 0+e],c2);patch([0 0 1 1-e 0+e 0+e],[0 1 1 1-e 1-e 0+e],c3);plot([0 1 1 0 0],[0 0 1 1 0]);disp('Mux');
  dotprod1 : neural/Weight Functions/dotprod
  "lz{4,3}" : Outport
      mask Display: e = 0.06;c1 = [120 230 180]/255;c2 = ([120 230 180]+0)/(256+128);c3 = ([120 230 180]+128)/(256+128);patch([0 1 1 0],[0 0 1 1],c1);patch([0 1 1 1-e 1-e 0+e],[0 0 1 1-e 0+e 0+e],c2);patch([0 0 1 1-e 0+e 0+e],[0 1 1 1-e 1-e 0+e],c3);plot([0 1 1 0 0],[0 0 1 1 0]);
  wires:
  "IW{4,3}(1,:)'"/1 -> dotprod1/1
  "ad{4,3}"/1 -> dotprod1/2
  dotprod1/1 -> Mux/1
  Mux/1 -> "lz{4,3}"/1

== matlab function state_space_all_model_reduce/CSI_Control_BIO/PQ_singlePhase ==
  data: va input; p output; vb input; ia input; ib input; q output
function [p, q] = fcn(va, vb, ia, ib)
% Esta funcion calcula la potencia activa y reactiva instantanea
% para el caso mnosofasico. En la revision de 2 papers he observado
% que una manera de extender la teoria de potencia al caso monofasico
% es asumiendo la tension o corriente de una fase como la componente
% alpha y hacer un desfase de 90 grados para obtener una version
% artificial de beta.

paux=va*ia+vb*ib;
if(paux > 20e4)
    paux = 20e4;
end
if(paux < -20e4)
    paux = -20e-4;
end

p = paux/2; % potencia activa instantanea

qaux = vb*ia-va*ib;

if(qaux>20e4)
    qaux=20e4;
end
if(qaux<-20e4)
    qaux=-20e4;
end

q = qaux/2; % potencia reactiva instantanea

== matlab function state_space_all_model_reduce/MeasureNode_I2/MATLAB Function ==
  data: u1 input; y output; u2 input; y2 output; u3 input; u4 input
function [y,y2] = fcn(u1,u2,u3,u4)

if u3==1
    
    if (u1>=0.5*10 && u1<=0.6) || (u1>=2*1 && u1<=2.2)|| (u1>=1*10 && u1<=1.3)%u1>=1000
        y=u2+u2*0.15;
        y2=u2*0.15;
    else
        y = u2;
        y2=0;
        
    end
elseif u3==2
    if (u1>=0.5*1 && u1<=0.6) || (u1>=2*1 && u1<=2.2)|| (u1>=1*100 && u1<=1.3)
        y=u4;
        y2=0;
    else
        y = u2;
        y2=0;
    end
    
else
    y = u2;
    y2=0;
end

== matlab function state_space_all_model_reduce/MATLAB Function1 ==
  data: x_hat1 input; v1 output; x_hat2 input; x_hat3 input; x_hat4 input; ruo1 input; rol input
function v1 = fcn(x_hat1,x_hat2,x_hat3,x_hat4,ruo1,rol)

% yol=[u1 ; u2];
% ym=[ym1 ; ym2];
%  C1=[zeros(1,10) 1];
 C1=[0 0 0 1];
 v11=C1*(x_hat4-x_hat1)*ruo1*rol;
 v12=C1*(x_hat4-x_hat2)*ruo1*rol;
 v13=C1*(x_hat4-x_hat3)*ruo1*rol;
 
 v1=-(v11+v12+v13);

== matlab function state_space_all_model_reduce/CSI_Control_BIO1/PQ2Iab_PH1 ==
  data: Va input; Ia output; Vb input; p input; q input; Ib output
function [Ia, Ib] = fcn(Va, Vb, p, q)
%#codegen
% Ia=0;
% Ib=0;
% divide by zero protection
if(abs((Va^2+Vb^2))<=1000*eps(0))
    det = 1/eps(0);
else
    det = 1/(Va^2+Vb^2); % constante auxiliar
end
%det = 1/(Va^2+Vb^2);

Mat = det*[Va Vb; Vb -Va];

Iab = Mat*[2*p;2*q];

Iaaux = Iab(1);
Ibaux = Iab(2);

ilim=1e3;

if(Iaaux>ilim)
    Iaaux=ilim;
end
if(Iaaux<-ilim)
    Iaaux =-ilim;    
end

if(isnan(Iaaux))
    Iaaux=0;
end
%-----------------


if(Ibaux>ilim)
    Ibaux=ilim;
end
if(Ibaux<-ilim)
    Ibaux =-ilim;    
end

if(isnan(Ibaux))
    Ibaux=0;
end
%-----------------


Ia = Iaaux;
Ib = Ibaux;

== matlab function state_space_all_model_reduce/CSI_Control_BIO1/PQ_singlePhase ==
  data: va input; p output; vb input; ia input; ib input; q output
function [p, q] = fcn(va, vb, ia, ib)
% Esta funcion calcula la potencia activa y reactiva instantanea
% para el caso mnosofasico. En la revision de 2 papers he observado
% que una manera de extender la teoria de potencia al caso monofasico
% es asumiendo la tension o corriente de una fase como la componente
% alpha y hacer un desfase de 90 grados para obtener una version
% artificial de beta.

paux=va*ia+vb*ib;
if(paux > 20e4)
    paux = 20e4;
end
if(paux < -20e4)
    paux = -20e-4;
end

p = paux/2; % potencia activa instantanea

qaux = vb*ia-va*ib;

if(qaux>20e4)
    qaux=20e4;
end
if(qaux<-20e4)
    qaux=-20e4;
end

q = qaux/2; % potencia reactiva instantanea

== matlab function state_space_all_model_reduce/MATLAB Function3 ==
  data: w input; y output; torque input; potencia input
function y = fcn(w,torque,potencia)
%#codegen

y = w*torque*1000/potencia;

== matlab function state_space_all_model_reduce/MATLAB Function SOC  ==
  data: u input; y output
function y = fcn(u)

y = -0.03536*u+100;

== matlab function state_space_all_model_reduce/CSI_Control_BIO/PQ2Iab_PH1 ==
  data: Va input; Ia output; Vb input; p input; q input; Ib output
function [Ia, Ib] = fcn(Va, Vb, p, q)
%#codegen
% Ia=0;
% Ib=0;
% divide by zero protection
if(abs((Va^2+Vb^2))<=1000*eps(0))
    det = 1/eps(0);
else
    det = 1/(Va^2+Vb^2); % constante auxiliar
end
%det = 1/(Va^2+Vb^2);

Mat = det*[Va Vb; Vb -Va];

Iab = Mat*[2*p;2*q];

Iaaux = Iab(1);
Ibaux = Iab(2);

ilim=1e3;

if(Iaaux>ilim)
    Iaaux=ilim;
end
if(Iaaux<-ilim)
    Iaaux =-ilim;    
end

if(isnan(Iaaux))
    Iaaux=0;
end
%-----------------


if(Ibaux>ilim)
    Ibaux=ilim;
end
if(Ibaux<-ilim)
    Ibaux =-ilim;    
end

if(isnan(Ibaux))
    Ibaux=0;
end
%-----------------


Ia = Iaaux;
Ib = Ibaux;
